simulink model "PIDcascadeTuning"  (R2023a)
settings: Solver=VariableStepAuto  StartTime=0.0  StopTime=10  RelTol=1e-3
values from neighbouring files (symbols this model uses):
  b_p = 0.0314    [CascadePID.m]    (also in LQR.m; model_verif.m = 0.0114)
  b_w = 1/(T*I_r)    (= 0.000346638655462)    [CascadePID.m]    (also in LQR.m; model_verif.m = 0.000315333070556)
  I = 0.011    [CascadePID.m]    (also in LQR.m; model_verif.m = 0.012)
  I_r = (I+I_w)/(I*I_w)    (= 424.242424242)    [CascadePID.m]    (also in LQR.m; model_verif.m = 416.666666667)
  K = 0.597    [CascadePID.m]    (also in Identification_TF.m = X(1); LQR.m; cost_TF.m = ',num2str(K),'; model_verif.m)
  K_m = G*b_w    (= 2.59112394958)    [CascadePID.m]    (also in LQR.m; model_verif.m = 2.3571147024)
undefined symbols (not defined in the file or in its folder): K_lqr
libraries: simulink x1
settings Model: Creator=claraneuburger  LastModifiedBy=claraneuburger

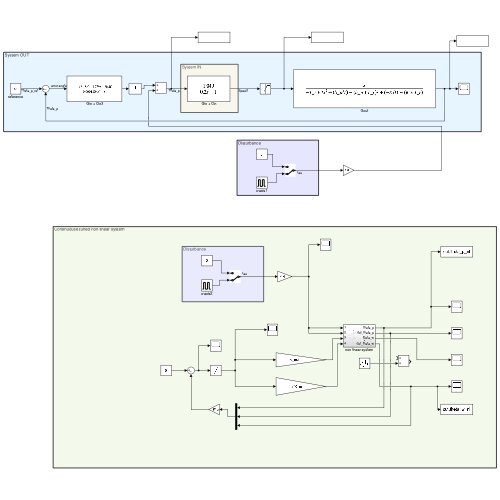
[thumbnail: Simulink's stored preview of the top-level diagram]
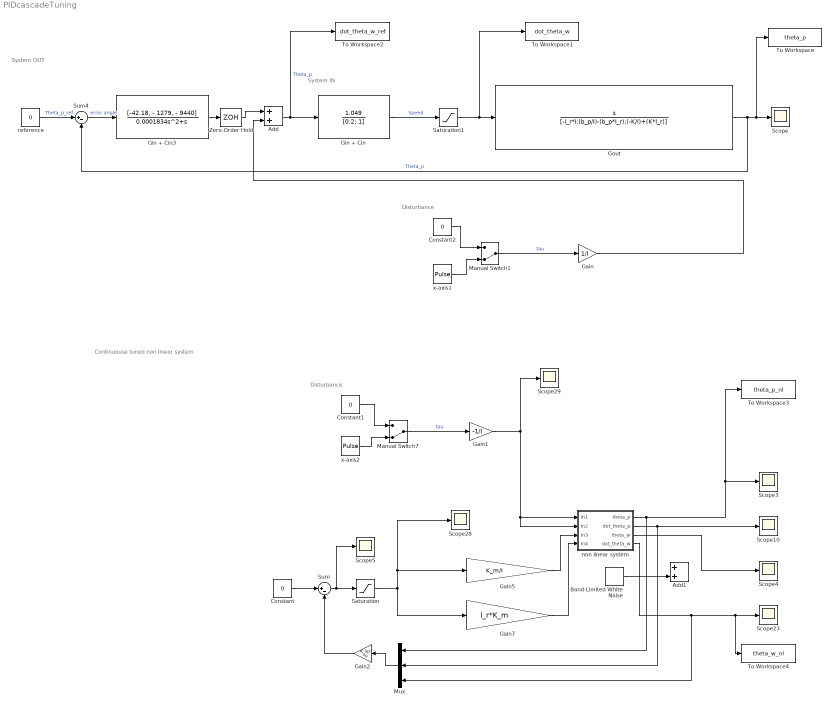
== system PIDcascadeTuning ==
  note: System OUT
  note: Disturbance
  note: System IN
  note: Continuouse tuned non linear system
  note: Disturbance
  " Gin + Cin" : TransferFcn  Numerator=[1.049]  Denominator=[0.2; 1]
  " Gin + Cin3" : TransferFcn  Numerator=[-42.18, - 1279, - 9440]  Denominator=[0.0001834,1,0]
  Add : Sum
  Add1 : Sum
  Band-Limited White Noise : simulink/Sources/Band-Limited White Noise  Cov=[0.3]  Ts=0.001  seed=[23341]
  Constant : Constant  Value=0
  Constant1 : Constant  Value=0
  Constant2 : Constant  Value=0
  Gain : Gain  Gain=1/I
  Gain1 : Gain  Gain=-1/I
  Gain2 : Gain  Gain=K_lqr  Multiplication=Matrix(K*u)
  Gain5 : Gain  Gain=K_m/I
  Gain7 : Gain  Gain=I_r*K_m
  Gout : TransferFcn  Numerator=[1 0]  Denominator=[-I_r*I;(b_p/I)-(b_p*I_r);(-K/I)+(K*I_r)]
  Manual Switch1 : ManualSwitch  CurrentSetting=0
  Manual Switch7 : ManualSwitch  CurrentSetting=0
  Mux : Mux  Inputs=3
  Saturation : Saturate  UpperLimit=2.33  LowerLimit=-2.33
  Saturation1 : Saturate  UpperLimit=5000  LowerLimit=-5000
  Scope{,3..5,10,23,28..29} (8 alike) : Scope
  Sum : Sum  Inputs=|+-
  Sum4 : Sum  Inputs=|+-
  To Workspace : ToWorkspace  VariableName=theta_p  SaveFormat=Timeseries  SampleTime=-1
  To Workspace1 : ToWorkspace  VariableName=dot_theta_w  SaveFormat=Timeseries  SampleTime=-1
  To Workspace2 : ToWorkspace  VariableName=dot_theta_w_ref  SaveFormat=Timeseries  SampleTime=-1
  To Workspace3 : ToWorkspace  VariableName=theta_p_nl  SaveFormat=Timeseries  SampleTime=-1
  To Workspace4 : ToWorkspace  VariableName=theta_w_nl  SaveFormat=Timeseries  SampleTime=-1
  Zero-Order Hold : ZeroOrderHold  SampleTime=0.01
  non linear system : Subsystem
  reference : Constant  Value=0
  x-axis1 : DiscretePulseGenerator  PulseType=Time based  Amplitude=100  Period=17  PulseWidth=0.01  PhaseDelay=1
  x-axis2 : DiscretePulseGenerator  PulseType=Time based  Amplitude=100  Period=17  PulseWidth=0.01  PhaseDelay=1
  wires:
  Sum4/1 -> " Gin + Cin3"/1  "error angle"
  " Gin + Cin"/1 -> Saturation1/1  "Speed"
  Manual Switch1/1 -> Gain/1  "tau"
  reference/1 -> Sum4/1  "Theta_p_ref"
  Saturation1/1 -> To Workspace1/1, Gout/1
  Constant2/1 -> Manual Switch1/1
  Gout/1 -> To Workspace/1, Scope/1, Sum4/2  "Theta_p"
  x-axis1/1 -> Manual Switch1/2
  Zero-Order Hold/1 -> Add/1
  Constant1/1 -> Manual Switch7/1
  Band-Limited White Noise/1 -> Add1/2
  Gain5/1 -> non linear system/3(In3)
  non linear system/2(dot_theta_p) -> Scope10/1, Mux/2
  Sum/1 -> Scope5/1, Saturation/1
  Gain1/1 -> Scope29/1, non linear system/2(In2), non linear system/1(In1)
  Gain2/1 -> Sum/2
  Constant/1 -> Sum/1
  Manual Switch7/1 -> Gain1/1  "tau"
  non linear system/1(theta_p) -> Mux/1, To Workspace3/1, Scope3/1
  Mux/1 -> Gain2/1
  Saturation/1 -> Gain7/1, Gain5/1, Scope28/1
  Gain7/1 -> non linear system/4(In4)
  non linear system/4(dot_theta_w) -> Mux/3, To Workspace4/1, Scope23/1
  non linear system/3(theta_w) -> Scope4/1
  x-axis2/1 -> Manual Switch7/2
  Gain/1 -> Add/2
  Add/1 -> To Workspace2/1, " Gin + Cin"/1  "Theta_p"
  " Gin + Cin3"/1 -> Zero-Order Hold/1

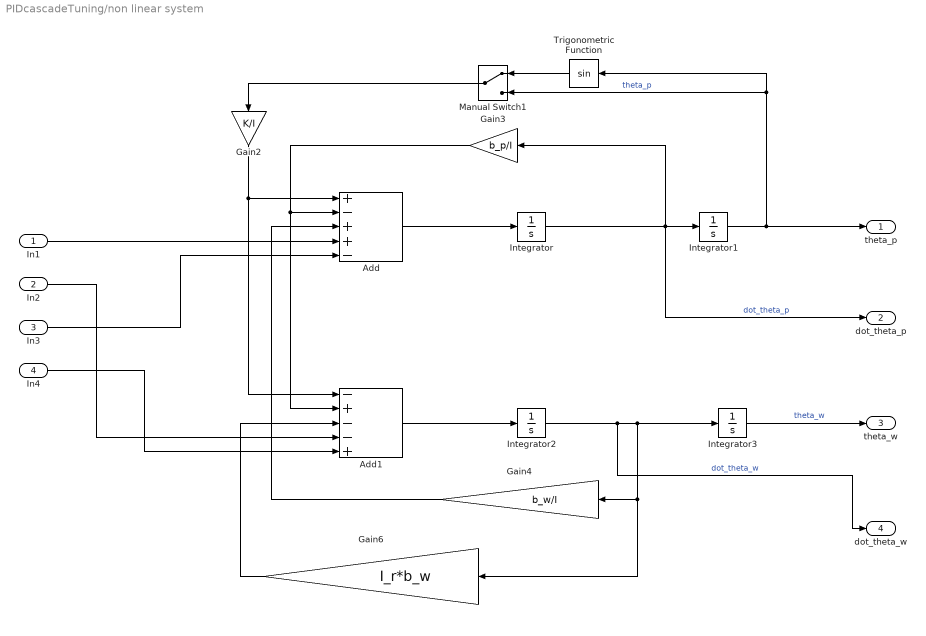
== system PIDcascadeTuning/non linear system ==
  In1 : Inport
  In2 : Inport  Port=2
  In3 : Inport  Port=3
  In4 : Inport  Port=4
  Add : Sum  Inputs=+-++-
  Add1 : Sum  Inputs=-+--+
  Gain2 : Gain  Gain=K/I
  Gain3 : Gain  Gain=b_p/I
  Gain4 : Gain  Gain=b_w/I
  Gain6 : Gain  Gain=I_r*b_w
  Integrator{,1..3} (4 alike) : Integrator
  Manual Switch1 : ManualSwitch
  Trigonometric Function : Trigonometry
  theta_p : Outport
  dot_theta_p : Outport  Port=2
  theta_w : Outport  Port=3
  dot_theta_w : Outport  Port=4
  wires:
  In2/1 -> Add1/4
  Gain6/1 -> Add1/3
  Integrator/1 -> dot_theta_p/1, Gain3/1, Integrator1/1  "dot_theta_p"
  Integrator2/1 -> Integrator3/1, Gain6/1, Gain4/1, dot_theta_w/1  "dot_theta_w"
  Gain4/1 -> Add/3
  Integrator1/1 -> theta_p/1, Manual Switch1/2, Trigonometric Function/1  "theta_p"
  Manual Switch1/1 -> Gain2/1
  In1/1 -> Add/4
  Gain2/1 -> Add1/1, Add/1
  Integrator3/1 -> theta_w/1  "theta_w"
  Add1/1 -> Integrator2/1
  Trigonometric Function/1 -> Manual Switch1/1
  In3/1 -> Add/5
  Add/1 -> Integrator/1
  In4/1 -> Add1/5
  Gain3/1 -> Add1/2, Add/2
